simulink model "GalvoModel_servolike_v2_simpli_B2"  (R2013a)
settings: Solver=ode45  StartTime=0.0  StopTime=10.0  RelTol=1e-3
values from neighbouring files (symbols this model uses):
  BEM = 108e-6    (= 0.000108)    [GalvoModel_thesis2_proc.m]
  CL = 180e-6    (= 0.00018)    [GalvoModel_thesis2_proc.m]    (also in GalvoModel_v4_sys.m = @(x,n) repmat(x, 1, n))
  CR = 2.79    [GalvoModel_thesis2_proc.m]
  FR = 4e-6    (= 4e-06)    [GalvoModel_thesis2_proc.m]
  KTR = 47e-3    (= 0.047)    [GalvoModel_thesis2_proc.m]
  RIN = 1.25e-8    (= 1.25e-08)    [GalvoModel_thesis2_proc.m]
  TRC = 6.17e-3    (= 0.00617)    [GalvoModel_thesis2_proc.m]
settings Model: Creator=mainster  LastModifiedBy=mainster
settings DebuggingCC: SolverPrmCheckMsg=none  InitInArrayFormatMsg=none

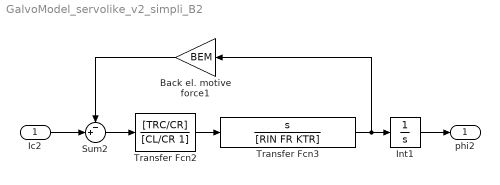
== system GalvoModel_servolike_v2_simpli_B2 ==
  Ic2 : Inport
  Back el. motive force1 : Gain  Gain=BEM
  Int1 : Integrator
  Sum2 : Sum  Inputs=-+|
  Transfer Fcn2 : TransferFcn  Numerator=[TRC/CR]  Denominator=[CL/CR 1]
  Transfer Fcn3 : TransferFcn  Numerator="[1  0]"  Denominator=[RIN FR KTR]
  phi2 : Outport
  wires:
  Ic2/1 -> Sum2/2
  Sum2/1 -> Transfer Fcn2/1
  Transfer Fcn3/1 -> Int1/1, Back el. motive force1/1
  Int1/1 -> phi2/1
  Back el. motive force1/1 -> Sum2/1
  Transfer Fcn2/1 -> Transfer Fcn3/1
